simulink model "TCM_controls"  (Simulink 8.1)
settings: Solver=ode45  StartTime=0.0  StopTime=10.0  RelTol=1e-3
undefined symbols (not defined in the file): bias, sgn, sigbuilder_block, sldvsubsys, StatesInp
libraries: simulink x4, sldvlib x1
(part 2 of 2)

== system TCM_controls/Controls/Signal Builder ==
  Demux : Demux  Tag=STV Demux  RequirementInfo={} %GIDa_5678e33d_a409_4daf_8a3c_a7653762ed72  Outputs=3
  FromWs : FromWorkspace  Tag=STV FromWs  RequirementInfo={} %GIDa_c232ff97_3303_4eed_9d83_58c8d1a3fdf2  VariableName=tuvar  SampleTime=0  SigBuilderData=DataTag16  VnvData=DataTag17
      SigBuilderData=|
      | common.afterFinalStr = 'Extrapolate'
      | common.sampleTime = 0
      | dataSet.timeRange = [0 60]
      | dataSet.name = 'Group 1'
      | sbobj.Groups.Name = 'Group 1'
      | sbobj.Groups.Signals(1).Name = 'Signal 1'
      | sbobj.Groups.Signals(1).XData = [0 1 1 60]
      | sbobj.Groups.Signals(1).YData = [0 0 30 30]
      | sbobj.Groups.Signals(2).Name = 'Signal 2'
      | sbobj.Groups.Signals(2).XData = [0 1 1 60]
      | sbobj.Groups.Signals(2).YData = [0 0 50 50]
      | sbobj.Groups.Signals(3).Name = 'Signal 3'
      | sbobj.Groups.Signals(3).XData = [0 1 1 60]
      | sbobj.Groups.Signals(3).YData = [0 0 90 90]
  Signal 1 : Outport  Tag=STV Outport  RequirementInfo={} %GIDa_8a7c9959_3ab1_4fa3_9237_02002c578c3a
  Signal 2 : Outport  Tag=STV Outport  RequirementInfo={} %GIDa_8214e080_4bbd_497a_a8e0_2403aa3353d6  Port=2
  Signal 3 : Outport  Tag=STV Outport  RequirementInfo={} %GIDa_d67e055c_1e4d_4845_80ff_06585dfc8bc5  Port=3
  wires:
  Demux/1 -> Signal 1/1
  FromWs/1 -> Demux/1
  Demux/2 -> Signal 2/1
  Demux/3 -> Signal 3/1

== system TCM_controls/Controls/Stall Protect ==
  In1 : Inport  RequirementInfo={} %GIDa_b580ff7f_a2a4_4d64_a593_e024c7b434b9
  Out1 : Outport  RequirementInfo={} %GIDa_c7daaf15_081b_46a4_b39b_dfa9229ab27b
  wires:
  In1/1 -> Out1/1

== system TCM_controls/Controls/Yaw Damper ==
  rdeg : Inport  RequirementInfo={} %GIDa_b24522de_e69b_48de_9af9_2692132d75e3
  CAS : Inport  RequirementInfo={} %GIDa_9040e143_9b5a_4bd4_9b3d_c7864ca39d4b  Port=2
  Kcas : Lookup  RequirementInfo={} %GIDa_605ad81f_30e9_4fb5_8ca6_c77de453bcbf  InputValues=[0 120 350 500]  Table=[1.0 1.0 0.3 0.3]
  Kr : Gain  RequirementInfo={} %GIDa_3271eca6_9d76_4a4e_a63b_379b60fbc601  Gain=1.25
  Product : Product  RequirementInfo={} %GIDa_62269e97_6254_4e35_a9a8_d83600cc999a  RndMeth=Zero
  YD_wo : TransferFcn  RequirementInfo={} %GIDa_4ac92844_e143_4f33_8651_adc16bd2d000  Numerator=[1 0]  Denominator=[1 10]
  RudCmd : Outport  RequirementInfo={} %GIDa_a1a869f2_e389_4b7c_a8e7_b9bd422cc732
  wires:
  rdeg/1 -> Kr/1
  CAS/1 -> Kcas/1
  Kcas/1 -> Product/2
  Product/1 -> RudCmd/1
  Kr/1 -> YD_wo/1
  YD_wo/1 -> Product/1

== system TCM_controls/Controls/Altitude Control/Safety Properties ==
  note: If altitude>100000 feets, deploy cannot be true.
  deploy : Inport  RequirementInfo={} %GIDa_dfcede91_9124_42cd_abbe_7ead53a64ff9
  altitude : Inport  RequirementInfo={} %GIDa_50687bca_593a_435a_8f31_14b7e665ff34  Port=2
  Compare To Constant : simulink/Logic and Bit Operations/Compare To Constant  RequirementInfo={} %GIDa_3f7a537f_9182_47f8_bcd5_ab4c14681b4e  relop=>  const=100000  OutDataTypeStr=uint8  ZeroCross=off
  Implies : sldvlib/Verification Utilities/Implies  RequirementInfo={} %GIDa_1e4cf76e_daba_4808_8bdd_5f375c017f16
  altitude valid : Assertion  RequirementInfo={} %GIDa_465ddf2e_4275_4b86_9045_34bd55a0fa0f
  wires:
  Implies/1 -> altitude valid/1
  Compare To Constant/1 -> Implies/1
  deploy/1 -> Implies/2
  altitude/1 -> Compare To Constant/1

== system TCM_controls/Controls/Altitude Control/Variable  Rate Limit ==
  ratelim : Inport  RequirementInfo={} %GIDa_d8223957_0ee6_4d0f_896d_927ffa49ae45
  input : Inport  RequirementInfo={} %GIDa_76bdf49d_0e81_4e96_831b_13498fa7c52f  Port=2
  ICtrig : Inport  RequirementInfo={} %GIDa_39ff20cc_57c8_4c35_9e5d_34015dc12136  Port=3
  IC : Inport  RequirementInfo={} %GIDa_2ce75480_2499_4122_a742_2b2b4edb9793  Port=4
  Gain : Gain  RequirementInfo={} %GIDa_d8b9db11_ed2f_4049_bd91_a49b0b010520  Gain=20  SaturateOnIntegerOverflow=on  OutDataTypeStr=Inherit: Same as input  ParamDataTypeStr=Inherit: Same as input
  Gain1 : Gain  RequirementInfo={} %GIDa_2fb03f98_a02f_456c_8989_01980bd546db  Gain=-1  SaturateOnIntegerOverflow=on  OutDataTypeStr=Inherit: Same as input  ParamDataTypeStr=Inherit: Same as input
  Integrator : Integrator  RequirementInfo={} %GIDa_51c88b5e_3fbc_400b_9a5f_59263bfd6f6e  ExternalReset=level  InitialConditionSource=external  IgnoreLimit=on
  Sum2 : Sum  RequirementInfo={} %GIDa_22614544_1142_4144_9dd9_aa039b4a2181  Inputs=|+-  SaturateOnIntegerOverflow=on
  Variable Limit Saturation : Subsystem  RequirementInfo={} %GIDa_286f79da_3fe7_4daf_8b5c_a86327e75d12
  output : Outport  RequirementInfo={} %GIDa_29546ac2_ecd4_4ec0_a107_b9bb2df4cf8f
  wires:
  Sum2/1 -> Gain/1
  Gain/1 -> Variable Limit Saturation/2(SigIn)
  ratelim/1 -> Gain1/1, Variable Limit Saturation/1(up_lim)
  Gain1/1 -> Variable Limit Saturation/3(Lo_lim)
  Variable Limit Saturation/1(Out1) -> Integrator/1
  Integrator/1 -> Sum2/2, output/1
  input/1 -> Sum2/1
  ICtrig/1 -> Integrator/2
  IC/1 -> Integrator/3

== system TCM_controls/Controls/Altitude Control/Variable Limit Saturation ==
  up_lim : Inport  RequirementInfo={} %GIDa_77c1c32c_801b_4b52_8276_d8decf959ab6
  SigIn : Inport  RequirementInfo={} %GIDa_ba6fd03f_651d_4873_8138_81e9e6db1fcd  Port=2
  Lo_lim : Inport  RequirementInfo={} %GIDa_b0ca3bb1_e016_41a3_85ee_6441aae5a6b1  Port=3
  Enforce low lim : MinMax  RequirementInfo={} %GIDa_e20ff77c_ec70_4c8a_beae_8e27e5cee3a6  Function=max  Inputs=2
  Enforce up lim : MinMax  RequirementInfo={} %GIDa_d194aa74_a596_49cd_bb83_16b9b32e9d4a  Inputs=2
  Out1 : Outport  RequirementInfo={} %GIDa_d13a4a43_a9c9_4c29_a62b_70fe5eabd527
  wires:
  Lo_lim/1 -> Enforce low lim/1
  SigIn/1 -> Enforce low lim/2
  Enforce low lim/1 -> Enforce up lim/1
  up_lim/1 -> Enforce up lim/2
  Enforce up lim/1 -> Out1/1

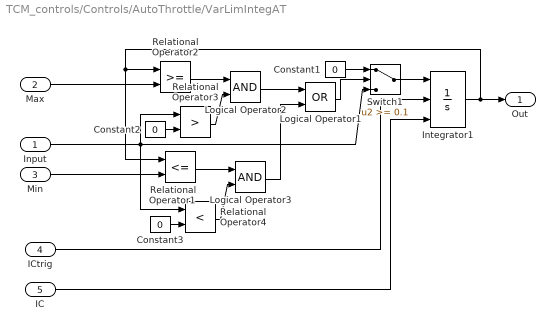
== system TCM_controls/Controls/AutoThrottle/VarLimIntegAT ==
  Input : Inport  RequirementInfo={} %GIDa_5b4ebf1a_bbef_4dad_995c_f852a36f584e
  Max : Inport  RequirementInfo={} %GIDa_00fa5381_d865_4287_abc2_f5622c7e0c9a  Port=2
  Min : Inport  RequirementInfo={} %GIDa_f7bb8f79_13a9_4bca_9cf8_e448736c46d1  Port=3
  ICtrig : Inport  RequirementInfo={} %GIDa_b2d1d038_df85_4102_b138_342afac5e762  Port=4
  IC : Inport  RequirementInfo={} %GIDa_d7b227ce_1a6e_4938_a6c1_e78ca9eddb9e  Port=5
  Constant1 : Constant  RequirementInfo={} %GIDa_270cf8f3_267e_47b5_ae2b_fcbfa4318be1  Value=0  SampleTime=-1
  Constant2 : Constant  RequirementInfo={} %GIDa_d78df232_0823_4c88_ba98_210c254f2ab3  Value=0  SampleTime=-1
  Constant3 : Constant  RequirementInfo={} %GIDa_b68fcc91_0022_453c_9b01_3bbc237609db  Value=0  SampleTime=-1
  Integrator1 : Integrator  RequirementInfo={} %GIDa_e9e4c7e9_1566_402d_bdde_796d137b7148  ExternalReset=level  InitialConditionSource=external
  Logical Operator1 : Logic  RequirementInfo={} %GIDa_45a3a50e_a7dc_4b40_b975_6f134a49bebe  Operator=OR
  Logical Operator2 : Logic  RequirementInfo={} %GIDa_728b7e64_1481_4419_9829_82572d49e5b1
  Logical Operator3 : Logic  RequirementInfo={} %GIDa_67dedde5_41a8_4767_9ca8_e38b1f0d566f
  Relational Operator1 : RelationalOperator  RequirementInfo={} %GIDa_8c5dce34_0367_4f53_94ea_e753e57c673e  Operator=<=  InputSameDT=on
  Relational Operator2 : RelationalOperator  RequirementInfo={} %GIDa_eff904f5_fefb_4ad9_bbf7_be23fbab1d3e  InputSameDT=on
  Relational Operator3 : RelationalOperator  RequirementInfo={} %GIDa_2d2faafc_ec4c_41b7_bb26_f44c56194c3e  Operator=>  InputSameDT=on
  Relational Operator4 : RelationalOperator  RequirementInfo={} %GIDa_cd476dad_dc4f_43ee_87d2_636c4a6aa66d  Operator=<  InputSameDT=on
  Switch1 : Switch  RequirementInfo={} %GIDa_17590294_7d88_4c0b_9049_2c6dcacf1638  Threshold=0.1  SaturateOnIntegerOverflow=on  InputSameDT=on
  Out : Outport  RequirementInfo={} %GIDa_cabf23e7_bdcd_4796_ab2d_062501ebe9d2
  wires:
  IC/1 -> Integrator1/3
  ICtrig/1 -> Integrator1/2
  Min/1 -> Relational Operator1/2
  Max/1 -> Relational Operator2/2
  Constant3/1 -> Relational Operator4/2
  Input/1 -> Switch1/3, Relational Operator3/1, Relational Operator4/1
  Logical Operator3/1 -> Logical Operator1/2
  Relational Operator4/1 -> Logical Operator3/2
  Relational Operator1/1 -> Logical Operator3/1
  Constant2/1 -> Relational Operator3/2
  Logical Operator2/1 -> Logical Operator1/1
  Relational Operator3/1 -> Logical Operator2/2
  Relational Operator2/1 -> Logical Operator2/1
  Logical Operator1/1 -> Switch1/2
  Integrator1/1 -> Relational Operator2/1, Relational Operator1/1, Out/1
  Switch1/1 -> Integrator1/1
  Constant1/1 -> Switch1/1

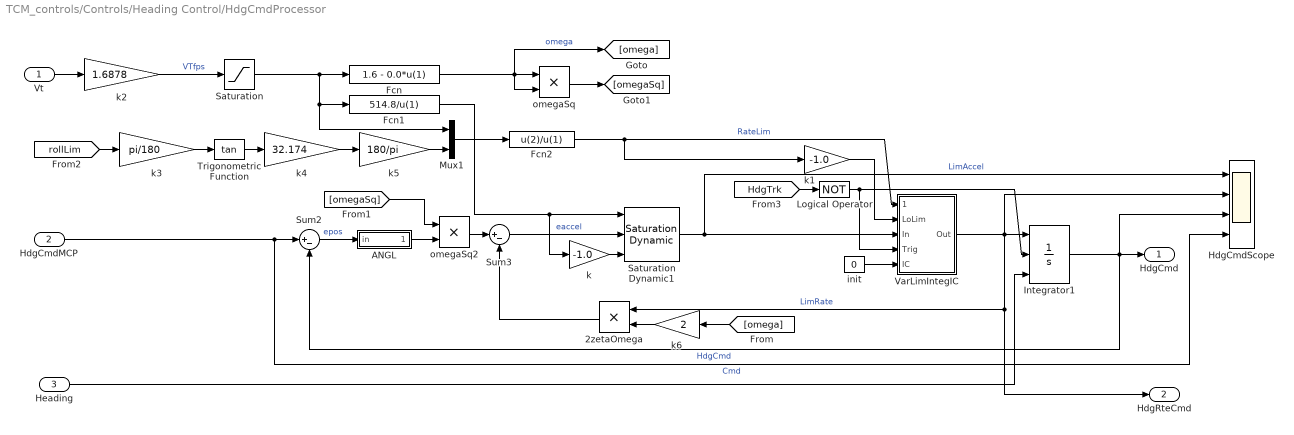
== system TCM_controls/Controls/Heading Control/HdgCmdProcessor ==
  Vt : Inport  RequirementInfo={} %GIDa_515ac05f_f942_4836_ace3_aea80432bda3
  HdgCmdMCP : Inport  RequirementInfo={} %GIDa_a61806b4_31e4_4af6_aba0_fd5c9dc0589c  Port=2
  Heading : Inport  RequirementInfo={} %GIDa_2567d72f_18a3_42c2_8f9e_9fc12c8f793b  Port=3
  2zetaOmega : Product  RequirementInfo={} %GIDa_c1462735_6161_4b0c_b463_31d6fa24eac6  RndMeth=Zero
  ANGL : Subsystem  RequirementInfo={} %GIDa_95577577_abd3_430d_afcd_cd4fd26c1c05
  Fcn : Fcn  RequirementInfo={} %GIDa_dcc0eba3_8613_4859_9538_b5893c431448  Expr=1.6 - 0.0*u(1)
  Fcn1 : Fcn  RequirementInfo={} %GIDa_3a21326f_238a_483f_8b28_742fa1dae0a9  Expr=514.8/u(1)
  Fcn2 : Fcn  RequirementInfo={} %GIDa_3531ad73_3344_4829_a511_797d1ae80842  Expr=u(2)/u(1)
  HdgCmdScope : Scope  NumInputPorts=4
      settings: RequirementInfo={} %GIDa_b0874fdc_2002_48b8_b18a_f40b0c866601  YMin=-2~-4~-40~-40  YMax=2~4~40~40  SaveName=ScopeData6
  Integrator1 : Integrator  RequirementInfo={} %GIDa_d74a792e_f737_4022_b760_0ef5c67ce78c  ExternalReset=level  InitialConditionSource=external
  Logical Operator : Logic  RequirementInfo={} %GIDa_6af60708_b902_47e8_901e_5265a3324604  Operator=NOT  AllPortsSameDT=off  OutDataTypeStr=boolean
  Mux1 : Mux  RequirementInfo={} %GIDa_5c9dab85_3a3e_4538_93a6_4586b9531d12  Inputs=2
  Saturation : Saturate  RequirementInfo={} %GIDa_5dbb8b75_efa9_49ab_9f9b_f6d22d37024f  UpperLimit=1000  LowerLimit=0.0001
  Saturation Dynamic1 : simulink/Discontinuities/Saturation Dynamic  RequirementInfo={} %GIDa_e3ee14ef_05d8_4d68_94dd_a3cea37f60a8  OutMin=[]  OutMax=[]  OutDataTypeStr=Inherit: Same as second input  OutDataType=fixdt(1, 16)  OutScaling=2^-10  DoSatur=off
  Sum2 : Sum  RequirementInfo={} %GIDa_dee77cac_e90e_467f_8b71_39ec4ee5fbe2  Inputs=|+-
  Sum3 : Sum  RequirementInfo={} %GIDa_e6e02489_2dcd_4397_aef4_351bd43f12bc  Inputs=|+-
  Trigonometric Function : Trigonometry  RequirementInfo={} %GIDa_63264a55_4968_4319_8a07_d9c9a78d4373  Operator=tan
  VarLimIntegIC : Subsystem  RequirementInfo={} %GIDa_ffa03bcd_b96e_4a19_93d8_e6c16918d833
  init : Constant  RequirementInfo={} %GIDa_ff7e49ee_25f0_4bf4_bb6d_16a2316c54f5  Value=0
  k : Gain  RequirementInfo={} %GIDa_436fd2c7_149a_4b79_9a7b_1f97517ce1d5  Gain=-1.0
  k1 : Gain  RequirementInfo={} %GIDa_e2bfec17_06ab_4d79_962d_6d451a8b3cff  Gain=-1.0
  k2 : Gain  RequirementInfo={} %GIDa_ee305c2a_0adf_4fc1_8f52_a40ece5cce4e  Gain=1.6878
  k3 : Gain  RequirementInfo={} %GIDa_baa8b95a_e3da_4d36_8033_b8346156e3d3  Gain=pi/180
  k4 : Gain  RequirementInfo={} %GIDa_1336b4d9_02ae_4ec5_8356_cde97dbcc1cf  Gain=32.174
  k5 : Gain  RequirementInfo={} %GIDa_2b28254a_5b2a_4423_ab50_2aa725a24fd7  Gain=180/pi
  k6 : Gain  RequirementInfo={} %GIDa_886988b4_6110_46ab_b9e8_ab309794bda7  Gain=2
  omegaSq : Product  RequirementInfo={} %GIDa_1c482a05_f7e7_4505_b94c_675969f793bb  RndMeth=Zero
  omegaSq2 : Product  RequirementInfo={} %GIDa_e36dcf3b_c5eb_45c9_a0ba_4e3316613325  RndMeth=Zero
  HdgCmd : Outport  RequirementInfo={} %GIDa_c73fb4c9_8875_40dc_ab51_899a73111f4e
  HdgRteCmd : Outport  RequirementInfo={} %GIDa_b44e6512_cb91_4f91_b3a8_a18b011d4db5  Port=2
  wires:
  Integrator1/1 -> Sum2/2, HdgCmd/1, HdgCmdScope/3  "HdgCmd"
  Vt/1 -> k2/1
  k2/1 -> Saturation/1  "VTfps"
  Fcn/1 -> omegaSq/2, omegaSq/1, [omega]  "omega"
  k/1 -> Saturation Dynamic1/3
  Mux1/1 -> Fcn2/1
  [rollLim] -> k3/1
  Sum3/1 -> Saturation Dynamic1/2  "eaccel"
  Saturation Dynamic1/1 -> VarLimIntegIC/3(In), HdgCmdScope/1  "LimAccel"
  k3/1 -> Trigonometric Function/1
  Trigonometric Function/1 -> k4/1
  k4/1 -> k5/1
  k5/1 -> Mux1/2
  Fcn2/1 -> VarLimIntegIC/1(UpLim), k1/1  "RateLim"
  k1/1 -> VarLimIntegIC/2(LoLim)
  VarLimIntegIC/1(Out) -> Integrator1/1, HdgCmdScope/2, 2zetaOmega/1, HdgRteCmd/1  "LimRate"
  [omega] -> k6/1
  k6/1 -> 2zetaOmega/2
  2zetaOmega/1 -> Sum3/2
  Fcn1/1 -> k/1, Saturation Dynamic1/1
  init/1 -> VarLimIntegIC/5(IC)
  [HdgTrk] -> Logical Operator/1
  omegaSq/1 -> [omegaSq]
  [omegaSq] -> omegaSq2/1
  omegaSq2/1 -> Sum3/1
  Sum2/1 -> ANGL/1(in)  "epos"
  HdgCmdMCP/1 -> Sum2/1, HdgCmdScope/4  "Cmd"
  ANGL/1(+ -180) -> omegaSq2/2
  Logical Operator/1 -> VarLimIntegIC/4(Trig), Integrator1/2
  Saturation/1 -> Fcn/1, Mux1/1, Fcn1/1
  Heading/1 -> Integrator1/3

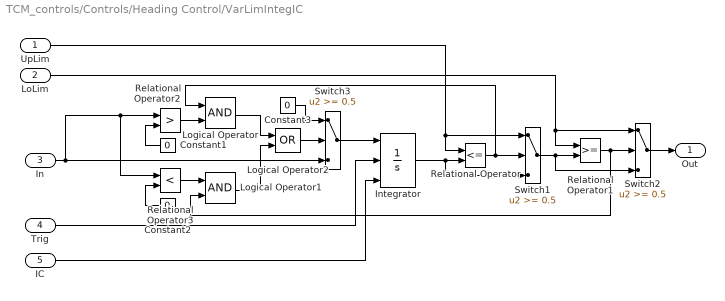
== system TCM_controls/Controls/Heading Control/VarLimIntegIC ==
  UpLim : Inport  RequirementInfo={} %GIDa_78d715a8_062e_4d46_9453_7068a7128550
  LoLim : Inport  RequirementInfo={} %GIDa_27698b44_41ff_4ef4_b81e_1083cedf5d48  Port=2
  In : Inport  RequirementInfo={} %GIDa_f8ed845c_d406_4181_95bd_d93b0570d058  Port=3
  Trig : Inport  RequirementInfo={} %GIDa_fd983cc5_6655_4fbd_9181_d2d047ebf916  Port=4
  IC : Inport  RequirementInfo={} %GIDa_af197525_76a4_40f3_8910_2319116cf4e3  Port=5
  Constant1 : Constant  RequirementInfo={} %GIDa_765eb5a9_e962_477a_b94d_22016d1144ca  Value=0
  Constant2 : Constant  RequirementInfo={} %GIDa_20e17dba_7a12_464c_ab69_a53f5fd5dede  Value=0
  Constant3 : Constant  RequirementInfo={} %GIDa_ca867b51_961f_4683_ac2c_df54bcef69cb  Value=0
  Integrator : Integrator  RequirementInfo={} %GIDa_04422ead_5b67_4bac_ac2a_3af71de67be4  ExternalReset=level  InitialConditionSource=external
  Logical Operator : Logic  RequirementInfo={} %GIDa_1188f909_ff31_4f00_9c86_62fde51e8e51  AllPortsSameDT=off
  Logical Operator1 : Logic  RequirementInfo={} %GIDa_f428af9f_6036_4525_9e89_505e4905906b  AllPortsSameDT=off
  Logical Operator2 : Logic  RequirementInfo={} %GIDa_4a1a0e80_aeec_4017_8d7b_db02fd2e0f49  Operator=OR  AllPortsSameDT=off
  Relational Operator : RelationalOperator  RequirementInfo={} %GIDa_4ba6cdf3_8a15_4323_8c30_b9c230aa673b  Operator=<=
  Relational Operator1 : RelationalOperator  RequirementInfo={} %GIDa_2248f585_9f4c_4fce_8dde_4b2890382944
  Relational Operator2 : RelationalOperator  RequirementInfo={} %GIDa_29f46b74_2a05_4486_a63e_005a0aa66144  Operator=>
  Relational Operator3 : RelationalOperator  RequirementInfo={} %GIDa_c274f1a5_58c8_4048_af99_f7ffdf739da4  Operator=<
  Switch1 : Switch  RequirementInfo={} %GIDa_cbc35896_a37d_404d_b7d2_f56df2af4d15  Threshold=0.5  SaturateOnIntegerOverflow=on  InputSameDT=on
  Switch2 : Switch  RequirementInfo={} %GIDa_a2473516_d298_46e6_8a3d_6016228f81ab  Threshold=0.5  SaturateOnIntegerOverflow=on  InputSameDT=on
  Switch3 : Switch  RequirementInfo={} %GIDa_8adafcda_6c55_4d53_ac6d_b95fe555805c  Threshold=0.5  SaturateOnIntegerOverflow=on  InputSameDT=on
  Out : Outport  RequirementInfo={} %GIDa_6a3c9b2e_9673_4734_8e2d_978a20063886
  wires:
  Relational Operator1/1 -> Logical Operator1/2, Switch2/2
  Switch1/1 -> Switch2/3, Relational Operator1/2
  LoLim/1 -> Relational Operator1/1, Switch2/1
  IC/1 -> Integrator/3
  Trig/1 -> Integrator/2
  Constant2/1 -> Relational Operator3/2
  Relational Operator3/1 -> Logical Operator1/1
  Logical Operator1/1 -> Logical Operator2/2
  Logical Operator/1 -> Logical Operator2/1
  Logical Operator2/1 -> Switch3/2
  Relational Operator2/1 -> Logical Operator/2
  Constant1/1 -> Relational Operator2/2
  In/1 -> Switch3/3, Relational Operator3/1, Relational Operator2/1
  Constant3/1 -> Switch3/1
  Switch3/1 -> Integrator/1
  Relational Operator/1 -> Logical Operator/1, Switch1/2
  Switch2/1 -> Out/1
  UpLim/1 -> Switch1/1, Relational Operator/1
  Integrator/1 -> Relational Operator/2, Switch1/3

== system TCM_controls/Controls/Manual Controls/Ail Command, deg ==
  Demux : Demux  Tag=STV Demux  RequirementInfo={} %GIDa_73d71eff_4db1_4242_ac47_12bfae37f36c  Outputs=1
  FromWs : FromWorkspace  Tag=STV FromWs  RequirementInfo={} %GIDa_a2a64bba_c280_49cc_822a_459b69ec6e7e  VariableName=tuvar  SampleTime=0  SigBuilderData=DataTag2  VnvData=DataTag3
      SigBuilderData=|
      | common.afterFinalStr = 'Extrapolate'
      | common.sampleTime = 0
      | dataSet.timeRange = [0 10]
      | dataSet.name = 'Group 1'
      | sbobj.Groups.Name = 'Group 1'
      | sbobj.Groups.Signals.Name = 'Doublet'
      | sbobj.Groups.Signals.XData = [0 1 1 2 2 2.98 2.98 10]
      | sbobj.Groups.Signals.YData = [0 0 5 5 -5 -5 0 0]
  Doublet : Outport  Tag=STV Outport  RequirementInfo={} %GIDa_4e93ace9_7a25_4b8f_86df_a4cd7da957c7
  wires:
  FromWs/1 -> Demux/1
  Demux/1 -> Doublet/1

== system TCM_controls/Controls/Manual Controls/Elev Command, deg ==
  Demux : Demux  Tag=STV Demux  RequirementInfo={} %GIDa_e2b6dd23_fe1d_4fb5_a45c_71d217965519  Outputs=2
  FromWs : FromWorkspace  Tag=STV FromWs  RequirementInfo={} %GIDa_90b4a387_db2f_4a71_b2ea_9105d995fffc  VariableName=tuvar  SampleTime=0  SigBuilderData=DataTag4  VnvData=DataTag5
      SigBuilderData=|
      | common.afterFinalStr = 'Extrapolate'
      | common.sampleTime = 0
      | dataSet.timeRange = [0 10]
      | dataSet.name = 'Group 1'
      | sbobj.Groups.Name = 'Group 1'
      | sbobj.Groups.Signals(1).Name = 'Doublet'
      | sbobj.Groups.Signals(1).XData = [0 1 1 2 2 3 3 10]
      | sbobj.Groups.Signals(1).YData = [0 0 5 5 -5 -5 0 0]
      | sbobj.Groups.Signals(2).Name = 'Pulse'
      | sbobj.Groups.Signals(2).XData = [0 1 1 2 2 10]
      | sbobj.Groups.Signals(2).YData = [0 0 1 1 0 0]
  Doublet : Outport  Tag=STV Outport  RequirementInfo={} %GIDa_9d87262d_6564_4396_800c_23677fddedb9
  Pulse : Outport  Tag=STV Outport  RequirementInfo={} %GIDa_8e7c0932_5a9f_47c8_a106_0355c9c5ab61  Port=2
  wires:
  Demux/1 -> Doublet/1
  FromWs/1 -> Demux/1
  Demux/2 -> Pulse/1

== system TCM_controls/Controls/Manual Controls/Rud Command, deg ==
  Demux : Demux  Tag=STV Demux  RequirementInfo={} %GIDa_20192c98_67fb_4f73_906a_554fcdd1b7ba  Outputs=2
  FromWs : FromWorkspace  Tag=STV FromWs  RequirementInfo={} %GIDa_46628748_e674_4377_b735_dd3dc4e6f360  VariableName=tuvar  SampleTime=0  SigBuilderData=DataTag6  VnvData=DataTag7
      SigBuilderData=|
      | common.afterFinalStr = 'Extrapolate'
      | common.sampleTime = 0
      | dataSet.timeRange = [0 10]
      | dataSet.name = 'Group 1'
      | sbobj.Groups.Name = 'Group 1'
      | sbobj.Groups.Signals(1).Name = 'Doublet'
      | sbobj.Groups.Signals(1).XData = [0 1 1 2 2 3 3 10]
      | sbobj.Groups.Signals(1).YData = [0 0 1 1 -1 -1 0 0]
      | sbobj.Groups.Signals(2).Name = 'Pulse'
      | sbobj.Groups.Signals(2).XData = [0 1 1 2 2 10]
      | sbobj.Groups.Signals(2).YData = [0 0 1 1 0 0]
  Doublet : Outport  Tag=STV Outport  RequirementInfo={} %GIDa_05262d29_ced2_47d7_bc0e_da54aa8a06eb
  Pulse : Outport  Tag=STV Outport  RequirementInfo={} %GIDa_7431bd65_25a5_485d_a83c_07d275f992b1  Port=2
  wires:
  Demux/1 -> Doublet/1
  FromWs/1 -> Demux/1
  Demux/2 -> Pulse/1

== system TCM_controls/Controls/Manual Controls/Throt Command, % ==
  Demux : Demux  Tag=STV Demux  RequirementInfo={} %GIDa_b6c9ce9b_63c3_42ef_95b4_91edc4a25592  Outputs=1
  FromWs : FromWorkspace  Tag=STV FromWs  RequirementInfo={} %GIDa_860afedb_09e0_45eb_8639_6581c3b2ac96  VariableName=tuvar  SampleTime=0  SigBuilderData=DataTag8  VnvData=DataTag9
      SigBuilderData=|
      | common.afterFinalStr = 'Extrapolate'
      | common.sampleTime = 0
      | dataSet.timeRange = [0 100]
      | dataSet.name = 'Group 1'
      | sbobj.Groups.Name = 'Group 1'
      | sbobj.Groups.Signals.Name = 'Pulse'
      | sbobj.Groups.Signals.XData = [0 5 5 90.2 90.2 100]
      | sbobj.Groups.Signals.YData = [0 0 1 1 0 0]
      | sbobj.Groups.TimeRange = [0 100]
  Pulse : Outport  Tag=STV Outport  RequirementInfo={} %GIDa_41d9af99_64dc_4e6c_969b_f91d6479ef21
  wires:
  FromWs/1 -> Demux/1
  Demux/1 -> Pulse/1

== system TCM_controls/Controls/ManualPitchcmd/Pitchcmd ==
  Demux : Demux  Tag=STV Demux  RequirementInfo={} %GIDa_8a64a477_6562_4cbf_bf0d_1714a1b3f865  Outputs=2
  FromWs : FromWorkspace  Tag=STV FromWs  RequirementInfo={} %GIDa_1ec4986b_bb17_487a_aa58_0c4c8a9f4c80  VariableName=tuvar  SampleTime=0  SigBuilderData=DataTag10  VnvData=DataTag11
      SigBuilderData=|
      | common.afterFinalStr = 'Extrapolate'
      | common.sampleTime = 0
      | dataSet.timeRange = [0 10]
      | dataSet.name = 'Group 1'
      | sbobj.Groups.Name = 'Group 1'
      | sbobj.Groups.Signals(1).Name = 'Signal 1'
      | sbobj.Groups.Signals(1).XData = [0 1 1 2 2 10]
      | sbobj.Groups.Signals(1).YData = [0 0 0.324 0.324 0 0]
      | sbobj.Groups.Signals(2).Name = 'Signal 2'
      | sbobj.Groups.Signals(2).XData = [0 1 1 1.1 1.1 10]
      | sbobj.Groups.Signals(2).YData = [0 0 1 1 0 0]
  Signal 1 : Outport  Tag=STV Outport  RequirementInfo={} %GIDa_7ec378dd_2e4e_4284_b478_1cb1bf86c202
  Signal 2 : Outport  Tag=STV Outport  RequirementInfo={} %GIDa_568e6ef2_3028_4676_a948_2f3b66cf34fa  Port=2
  wires:
  Demux/2 -> Signal 2/1
  Demux/1 -> Signal 1/1
  FromWs/1 -> Demux/1

== system TCM_controls/Controls/ManualRollcmd/Rollcmd ==
  Demux : Demux  Tag=STV Demux  RequirementInfo={} %GIDa_530dd108_d4a2_40a8_8374_11420e655f18  Outputs=2
  FromWs : FromWorkspace  Tag=STV FromWs  RequirementInfo={} %GIDa_17f71a9a_1247_4e75_8c43_acc8273bec58  VariableName=tuvar  SampleTime=0  SigBuilderData=DataTag12  VnvData=DataTag13
      SigBuilderData=|
      | common.afterFinalStr = 'Extrapolate'
      | common.sampleTime = 0
      | dataSet.timeRange = [0 10]
      | dataSet.name = 'Group 1'
      | sbobj.Groups.Name = 'Group 1'
      | sbobj.Groups.Signals(1).Name = 'Signal 1'
      | sbobj.Groups.Signals(1).XData = [0 1 1 2 2 10]
      | sbobj.Groups.Signals(1).YData = [0 0 0.324 0.324 0 0]
      | sbobj.Groups.Signals(2).Name = 'Signal 2'
      | sbobj.Groups.Signals(2).XData = [0 1 1 1.1 1.1 10]
      | sbobj.Groups.Signals(2).YData = [0 0 1 1 0 0]
  Signal 1 : Outport  Tag=STV Outport  RequirementInfo={} %GIDa_de19c236_7af2_41d2_90e9_823123dc628f
  Signal 2 : Outport  Tag=STV Outport  RequirementInfo={} %GIDa_47fb4f22_be31_440c_a25c_c311b550e5a2  Port=2
  wires:
  FromWs/1 -> Demux/1
  Demux/1 -> Signal 1/1
  Demux/2 -> Signal 2/1

== system TCM_controls/Controls/PitchCmd/Pitchcmd1 ==
  Demux : Demux  Tag=STV Demux  RequirementInfo={} %GIDa_64b8766b_969e_4944_94e8_48149aee3985  Outputs=1
  FromWs : FromWorkspace  Tag=STV FromWs  RequirementInfo={} %GIDa_70842ccc_6b40_4067_a172_866dc888187a  VariableName=tuvar  SampleTime=0  SigBuilderData=DataTag14  VnvData=DataTag15
      SigBuilderData=|
      | common.afterFinalStr = 'Extrapolate'
      | common.sampleTime = 0
      | dataSet.timeRange = [0 10]
      | dataSet.name = 'Group 1'
      | sbobj.Groups.Name = 'Group 1'
      | sbobj.Groups.Signals.Name = 'Signal 1'
      | sbobj.Groups.Signals.XData = [0 1 1 6 10]
      | sbobj.Groups.Signals.YData = [0 0 1 1 1]
  Signal 1 : Outport  Tag=STV Outport  RequirementInfo={} %GIDa_c80681f1_2732_4655_8557_843907e9d24b
  wires:
  FromWs/1 -> Demux/1
  Demux/1 -> Signal 1/1

== system TCM_controls/Controls/Altitude Control/Variable  Rate Limit/Variable Limit Saturation ==
  up_lim : Inport  RequirementInfo={} %GIDa_0d53a3c4_d793_4e99_8ec6_92d253e67af3
  SigIn : Inport  RequirementInfo={} %GIDa_26772f44_fc63_45ef_9688_e7cf5f1fbe53  Port=2
  Lo_lim : Inport  RequirementInfo={} %GIDa_4c9a2420_a2ae_46d5_b438_96108cb59fe8  Port=3
  Enforce low lim : MinMax  RequirementInfo={} %GIDa_561b8c33_8acc_47cd_8096_b3556837cd6b  Function=max  Inputs=2
  Enforce up lim : MinMax  RequirementInfo={} %GIDa_86fd5ae4_a39a_44da_abc4_c95665abb6bb  Inputs=2
  Out1 : Outport  RequirementInfo={} %GIDa_645eb44c_926a_4d04_a11d_68f755032eb6
  wires:
  Enforce up lim/1 -> Out1/1
  up_lim/1 -> Enforce up lim/2
  Enforce low lim/1 -> Enforce up lim/1
  SigIn/1 -> Enforce low lim/2
  Lo_lim/1 -> Enforce low lim/1

== system TCM_controls/Controls/Heading Control/HdgCmdProcessor/ANGL ==
  in : Inport  RequirementInfo={} %GIDa_6d7c8d47_537b_4461_ba54_f42dc27779ac
  Constant1 : Constant  RequirementInfo={} %GIDa_8f36dbca_67ec_405e_9355_0577880a4bb8  Value=180
  Fcn1 : Fcn  RequirementInfo={} %GIDa_75118b4f_0a86_42cb_86f0_b7de401330e2  Expr=360*sgn(u(1))
  Fcn2 : Fcn  RequirementInfo={} %GIDa_ca210c9e_26df_472b_81ad_06362d6b1453  Expr=abs(u(1))
  Relational Operator : RelationalOperator  RequirementInfo={} %GIDa_b79ec4ed_7255_48e6_8dec_3e080662da51  Operator=>
  Sum6 : Sum  RequirementInfo={} %GIDa_a6c73a7c_eaef_41b5_b487_fe214ea9fb62  Inputs=|-+  SaturateOnIntegerOverflow=on
  Switch1 : Switch  RequirementInfo={} %GIDa_c9dd3e65_cef9_4045_b1f6_87551a037bc7  Threshold=0.1  SaturateOnIntegerOverflow=on
  + -180 : Outport  RequirementInfo={} %GIDa_6113f85c_6408_4f19_8155_832842520110
  wires:
  Fcn2/1 -> Relational Operator/1
  in/1 -> Switch1/3, Sum6/2, Fcn1/1, Fcn2/1
  Switch1/1 -> + -180/1
  Fcn1/1 -> Sum6/1
  Sum6/1 -> Switch1/1
  Relational Operator/1 -> Switch1/2
  Constant1/1 -> Relational Operator/2

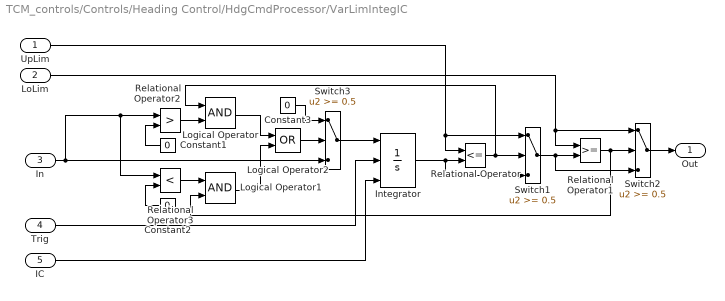
== system TCM_controls/Controls/Heading Control/HdgCmdProcessor/VarLimIntegIC ==
  UpLim : Inport  RequirementInfo={} %GIDa_d1df2537_54c6_4759_81e5_dbeb6e8aa58f
  LoLim : Inport  RequirementInfo={} %GIDa_fdd79fb2_838d_415d_8368_833fc34fed37  Port=2
  In : Inport  RequirementInfo={} %GIDa_022e1d3e_87f9_4e81_a830_b4381791aeb8  Port=3
  Trig : Inport  RequirementInfo={} %GIDa_9f1979fe_9f13_4b95_a2e8_fb9f68d2a399  Port=4
  IC : Inport  RequirementInfo={} %GIDa_b2939014_df20_41e4_b38d_5085018aaba2  Port=5
  Constant1 : Constant  RequirementInfo={} %GIDa_331b65bb_5823_45e2_ba13_fee3f6cb192f  Value=0
  Constant2 : Constant  RequirementInfo={} %GIDa_2e1cd29b_791b_474b_8c61_05f63dc07bd0  Value=0
  Constant3 : Constant  RequirementInfo={} %GIDa_58022a98_2ad4_4a1e_a9c8_99034c2d751b  Value=0
  Integrator : Integrator  RequirementInfo={} %GIDa_b3fd41f5_414b_4b86_8ca5_d8f4fdd3d64f  ExternalReset=level  InitialConditionSource=external
  Logical Operator : Logic  RequirementInfo={} %GIDa_c2d47470_c4e2_40a9_97a5_e9dd484b3ea1  AllPortsSameDT=off
  Logical Operator1 : Logic  RequirementInfo={} %GIDa_dff133a9_0880_44fa_818f_22184b3cbccb  AllPortsSameDT=off
  Logical Operator2 : Logic  RequirementInfo={} %GIDa_f5fe9366_8578_492e_9bee_789c9667baba  Operator=OR  AllPortsSameDT=off
  Relational Operator : RelationalOperator  RequirementInfo={} %GIDa_391a2f2a_0b80_48a0_95b5_cc0204fd51ec  Operator=<=
  Relational Operator1 : RelationalOperator  RequirementInfo={} %GIDa_9fb4107e_63a0_4e79_852a_8e6895b75b3d
  Relational Operator2 : RelationalOperator  RequirementInfo={} %GIDa_da08b36f_63f8_42dd_a794_cedac9ae66e7  Operator=>
  Relational Operator3 : RelationalOperator  RequirementInfo={} %GIDa_9355ee96_6bb9_4fd6_859f_0d0d83f8523e  Operator=<
  Switch1 : Switch  RequirementInfo={} %GIDa_7b0c6a26_bc23_4c6e_a4f2_3b024d78c908  Threshold=0.5  SaturateOnIntegerOverflow=on  InputSameDT=on
  Switch2 : Switch  RequirementInfo={} %GIDa_0edd32af_e210_47f0_903a_ff5c65a2acde  Threshold=0.5  SaturateOnIntegerOverflow=on  InputSameDT=on
  Switch3 : Switch  RequirementInfo={} %GIDa_b5ce6b35_c0da_4591_bcc6_3b2189dd3636  Threshold=0.5  SaturateOnIntegerOverflow=on  InputSameDT=on
  Out : Outport  RequirementInfo={} %GIDa_408823de_88fe_4388_93be_562b6a6573e6
  wires:
  Relational Operator1/1 -> Logical Operator1/2, Switch2/2
  Switch1/1 -> Switch2/3, Relational Operator1/2
  LoLim/1 -> Relational Operator1/1, Switch2/1
  IC/1 -> Integrator/3
  Trig/1 -> Integrator/2
  Constant2/1 -> Relational Operator3/2
  Relational Operator3/1 -> Logical Operator1/1
  Logical Operator1/1 -> Logical Operator2/2
  Logical Operator/1 -> Logical Operator2/1
  Logical Operator2/1 -> Switch3/2
  Relational Operator2/1 -> Logical Operator/2
  Constant1/1 -> Relational Operator2/2
  In/1 -> Switch3/3, Relational Operator3/1, Relational Operator2/1
  Constant3/1 -> Switch3/1
  Switch3/1 -> Integrator/1
  Relational Operator/1 -> Logical Operator/1, Switch1/2
  Switch2/1 -> Out/1
  UpLim/1 -> Switch1/1, Relational Operator/1
  Integrator/1 -> Relational Operator/2, Switch1/3
